simulink model "rmspec"  (Simulink 7.0)
settings: Solver=ode45  StartTime=0.0  StopTime=200  RelTol=1e-3
undefined symbols (not defined in the file): pfb_coeff_gen_calc
libraries: xbsIndex_r4 x3092, casper_library x230, xps_library x24
(part 20 of 33)

== system rmspec/pfb/fft_wideband_real1/fft_direct/butterfly1_1/twiddle/coeff_gen ==
  rst : Inport
  Counter : xbsIndex_r4/Counter  cnt_type=Free Running  cnt_to=Inf  operation=Up  start_count=0  cnt_by_val=1  arith_type=Unsigned  n_bits=9  bin_pt=0  load_pin=off  rst=on  en=off  explicit_period=on  period=1  dbl_ovrd=off  use_behavioral_HDL=off  use_rpm=off  implementation=Fabric  block_type=counter
  ROM : xbsIndex_r4/ROM  depth=512  initVector=[1 0.999984741210938 0.999923706054688 0.999832153320313 0.999702453613281 0.999526977539063 0.999320983886719 0.999076843261719 0.998794555664063 0.99847412109375 0.998115539550781 0.997726440429688 0.997291564941406 0.996818542480469 0.996315002441406 0.995765686035156 0.995185852050781 0.99456787109375 0.993904113769531 0.993209838867188 0.992477416992188 0.991706848144531 0.99090576171875 0.990058898925781 0.989173889160156 0.988258361816406 0.9873046875 0.986305236816406 0.985275268554688 0.984207153320313 0.983108520507813 0.981964111328125 0.980781555175781 0.979568481445313 0.978317260742188 0.977027893066406 0.975700378417969 0.974342346191406 0.972938537597656 0.971504211425781 0.97003173828125 0.968521118164063 0.96697998046875 0.96539306640625 0.963775634765625 0.962120056152344 0.960433959960938 0.958702087402344 0.956939697265625 0.95513916015625 0.95330810546875 0.951431274414063 0.949531555175781 0.947586059570313 0.945610046386719 0.943595886230469 0.941543579101563 0.939460754394531 0.937339782714844 0.9351806640625 0.932991027832031 0.930763244628906 0.928504943847656 0.92620849609375 0.923881530761719 0.921516418457031 0.919113159179688 0.916679382324219 0.914207458496094 0.911705017089844 0.909164428710938 0.906593322753906 0.90399169921875 0.901351928710938 0.898674011230469 0.895965576171875 0.893226623535156 0.890449523925781 0.887641906738281 0.884796142578125 0.881919860839844 0.879013061523438 0.876068115234375 0.873092651367188 0.870086669921875 0.867042541503906 0.863975524902344 0.860870361328125 0.85772705078125 0.854560852050781 0.851356506347656 0.848121643066406 0.844856262207031 0.841552734375 0.838226318359375 0.834861755371094 0.831466674804688 0.828048706054688 0.824592590332031 0.82110595703125 0.817581176757813 0.814033508300781 0.810455322265625 0.806846618652344 0.803207397460938 0.799537658691406 0.79583740234375 0.792106628417969 0.788345336914063 0.784553527832031 0.780738830566406 0.776885986328125 0.77301025390625 0.76910400390625 0.765167236328125 0.761199951171875 0.757209777832031 0.753189086914063 0.749137878417969 0.74505615234375 0.740951538085938 0.73681640625 0.732650756835938 0.728462219238281 0.724250793457031 0.720001220703125 0.715728759765625 0.711433410644531 0.707107543945313 0.702751159667969 0.698379516601563 0.6939697265625 0.689537048339844 0.685081481933594 0.68060302734375 0.676094055175781 0.671562194824219 0.666999816894531 0.66241455078125 0.657806396484375 0.653175354003906 0.648513793945313 0.643829345703125 0.639122009277344 0.634391784667969 0.629638671875 0.624862670898438 0.62005615234375 0.615234375 0.610382080078125 0.605514526367188 0.600616455078125 0.595695495605469 0.59075927734375 0.585800170898438 0.580810546875 0.5758056640625 0.570777893066406 0.56573486328125 0.560661315917969 0.555572509765625 0.550460815429688 0.545326232910156 0.540168762207031 0.534996032714844 0.529800415039063 0.524589538574219 0.519355773925781 0.51409912109375 0.508827209472656 0.5035400390625 0.49822998046875 0.492897033691406 0.487548828125 0.482185363769531 0.476799011230469 0.471397399902344 0.465972900390625 0.460540771484375 0.455085754394531 0.449607849121094 0.444122314453125 0.438613891601563 0.433090209960938 0.427558898925781 0.4219970703125 0.416427612304688 0.410842895507813 0.405242919921875 0.399627685546875 0.393989562988281 0.388343811035156 0.382682800292969 0.377006530761719 0.371315002441406 0.365615844726563 0.359893798828125 0.354164123535156 0.348419189453125 0.342658996582031 0.336891174316406 0.331108093261719 0.325309753417969 0.319503784179688 0.313682556152344 0.307846069335938 0.302009582519531 0.296150207519531 0.290283203125 0.284408569335938 0.278518676757813 0.272621154785156 0.266716003417969 0.260795593261719 0.254867553710938 0.248924255371094 0.24298095703125 0.237022399902344 0.231056213378906 0.225082397460938 0.219100952148438 0.213111877441406 0.207115173339844 0.201103210449219 0.195091247558594 0.189071655273438 ...(+5321 chars)]  distributed_mem=Block RAM  rst=off  init_reg=0  en=off  latency=2  arith_type="Signed  (2's comp)"  n_bits=18  bin_pt=17  dbl_ovrd=off  optimize=Area  use_rpm=on  block_type=sprom
      settings: block_version=10.1.3
  ROM1 : xbsIndex_r4/ROM  depth=512  initVector=[0 -0.006134033203125 -0.01226806640625 -0.0184097290039063 -0.0245437622070313 -0.0306777954101563 -0.03680419921875 -0.042938232421875 -0.0490646362304688 -0.0551986694335938 -0.0613174438476563 -0.06744384765625 -0.0735626220703125 -0.079681396484375 -0.0858001708984375 -0.0919113159179688 -0.0980148315429688 -0.104118347167969 -0.110221862792969 -0.116317749023438 -0.122413635253906 -0.128501892089844 -0.13458251953125 -0.140655517578125 -0.146728515625 -0.152793884277344 -0.158859252929688 -0.164909362792969 -0.17095947265625 -0.177001953125 -0.183036804199219 -0.189071655273438 -0.195091247558594 -0.201103210449219 -0.207115173339844 -0.213111877441406 -0.219100952148438 -0.225082397460938 -0.231056213378906 -0.237022399902344 -0.24298095703125 -0.248924255371094 -0.254867553710938 -0.260795593261719 -0.266716003417969 -0.272621154785156 -0.278518676757813 -0.284408569335938 -0.290283203125 -0.296150207519531 -0.302009582519531 -0.307846069335938 -0.313682556152344 -0.319503784179688 -0.325309753417969 -0.331108093261719 -0.336891174316406 -0.342658996582031 -0.348419189453125 -0.354164123535156 -0.359893798828125 -0.365615844726563 -0.371315002441406 -0.377006530761719 -0.382682800292969 -0.388343811035156 -0.393989562988281 -0.399627685546875 -0.405242919921875 -0.410842895507813 -0.416427612304688 -0.4219970703125 -0.427558898925781 -0.433090209960938 -0.438613891601563 -0.444122314453125 -0.449607849121094 -0.455085754394531 -0.460540771484375 -0.465972900390625 -0.471397399902344 -0.476799011230469 -0.482185363769531 -0.487548828125 -0.492897033691406 -0.49822998046875 -0.5035400390625 -0.508827209472656 -0.51409912109375 -0.519355773925781 -0.524589538574219 -0.529800415039063 -0.534996032714844 -0.540168762207031 -0.545326232910156 -0.550460815429688 -0.555572509765625 -0.560661315917969 -0.56573486328125 -0.570777893066406 -0.5758056640625 -0.580810546875 -0.585800170898438 -0.59075927734375 -0.595695495605469 -0.600616455078125 -0.605514526367188 -0.610382080078125 -0.615234375 -0.62005615234375 -0.624862670898438 -0.629638671875 -0.634391784667969 -0.639122009277344 -0.643829345703125 -0.648513793945313 -0.653175354003906 -0.657806396484375 -0.66241455078125 -0.666999816894531 -0.671562194824219 -0.676094055175781 -0.68060302734375 -0.685081481933594 -0.689537048339844 -0.6939697265625 -0.698379516601563 -0.702751159667969 -0.707107543945313 -0.711433410644531 -0.715728759765625 -0.720001220703125 -0.724250793457031 -0.728462219238281 -0.732650756835938 -0.73681640625 -0.740951538085938 -0.74505615234375 -0.749137878417969 -0.753189086914063 -0.757209777832031 -0.761199951171875 -0.765167236328125 -0.76910400390625 -0.77301025390625 -0.776885986328125 -0.780738830566406 -0.784553527832031 -0.788345336914063 -0.792106628417969 -0.79583740234375 -0.799537658691406 -0.803207397460938 -0.806846618652344 -0.810455322265625 -0.814033508300781 -0.817581176757813 -0.82110595703125 -0.824592590332031 -0.828048706054688 -0.831466674804688 -0.834861755371094 -0.838226318359375 -0.841552734375 -0.844856262207031 -0.848121643066406 -0.851356506347656 -0.854560852050781 -0.85772705078125 -0.860870361328125 -0.863975524902344 -0.867042541503906 -0.870086669921875 -0.873092651367188 -0.876068115234375 -0.879013061523438 -0.881919860839844 -0.884796142578125 -0.887641906738281 -0.890449523925781 -0.893226623535156 -0.895965576171875 -0.898674011230469 -0.901351928710938 -0.90399169921875 -0.906593322753906 -0.909164428710938 -0.911705017089844 -0.914207458496094 -0.916679382324219 -0.919113159179688 -0.921516418457031 -0.923881530761719 -0.92620849609375 -0.928504943847656 -0.930763244628906 -0.932991027832031 -0.9351806640625 -0.937339782714844 -0.939460754394531 -0.941543579101563 -0.943595886230469 -0.945610046386719 -0.947586059570313 -0.949531555175781 -0.951431274414063 -0.95330810546875 -0.95513916015625 -0.956939697265625 -0.958702087402344 -0.960433959960938 -0.962120056152344 -0.963775634765625 -0.96539306640625 ...(+5571 chars)]  distributed_mem=Block RAM  rst=off  init_reg=0  en=off  latency=2  arith_type="Signed  (2's comp)"  n_bits=18  bin_pt=17  dbl_ovrd=off  optimize=Area  use_rpm=on  block_type=sprom
      settings: block_version=10.1.3
  Slice : xbsIndex_r4/Slice  nbits=9  boolean_output=off  mode=Upper Bit Location + Width  bit1=0  base1=MSB of Input  bit0=0  base0=LSB of Input  dbl_ovrd=off  block_type=slice
      settings: infoedit="Extracts a given range of bits from each input sample and presents it at the output.  The output type is ordinarily unsigned with binary point at zero, but can be Boolean when the slice is one bit wide.<P><P>Hardware notes: In hardware this block costs nothing."  block_version=10.1.3
  ri_to_c : casper_library/Misc/ri_to_c  SystemSampleTime=-1
  w : Outport
  wires:
  ri_to_c/1 -> w/1
  rst/1 -> Counter/1
  Counter/1 -> Slice/1
  Slice/1 -> ROM/1, ROM1/1
  ROM/1 -> ri_to_c/1
  ROM1/1 -> ri_to_c/2

== system rmspec/pfb/fft_wideband_real1/fft_direct/butterfly1_1/twiddle/convert_of ==
  din : Inport  OutDataType=sfix(16)  OutScaling=2^0
  convert : xbsIndex_r4/Convert  arith_type="Signed  (2's comp)"  n_bits=bit_width_o  bin_pt=binary_point_o  quantization=Truncate  overflow=Wrap  latency=latency  dbl_ovrd=off  pipeline=on  block_type=convert
      settings: block_version=10.1.1
  never : xbsIndex_r4/Constant  arith_type=Boolean  const=0  n_bits=16  bin_pt=14  explicit_period=on  period=1  equ=P=C  opselect=C  inp2=PCIN>>17  opr=+  inp1=P  carry=CIN  dbl_ovrd=off  block_type=constant
  dout : Outport
  of : Outport  Port=2
  wires:
  din/1 -> convert/1
  convert/1 -> dout/1
  never/1 -> of/1

== system rmspec/pfb/fft_wideband_real1/fft_direct/butterfly1_1/twiddle/convert_of1 ==
  din : Inport  OutDataType=sfix(16)  OutScaling=2^0
  convert : xbsIndex_r4/Convert  arith_type="Signed  (2's comp)"  n_bits=bit_width_o  bin_pt=binary_point_o  quantization=Truncate  overflow=Wrap  latency=latency  dbl_ovrd=off  pipeline=on  block_type=convert
      settings: block_version=10.1.1
  never : xbsIndex_r4/Constant  arith_type=Boolean  const=0  n_bits=16  bin_pt=14  explicit_period=on  period=1  equ=P=C  opselect=C  inp2=PCIN>>17  opr=+  inp1=P  carry=CIN  dbl_ovrd=off  block_type=constant
  dout : Outport
  of : Outport  Port=2
  wires:
  din/1 -> convert/1
  convert/1 -> dout/1
  never/1 -> of/1

== system rmspec/pfb/fft_wideband_real1/fft_direct/butterfly2_0/twiddle/coeff_gen ==
  rst : Inport
  Counter : xbsIndex_r4/Counter  cnt_type=Free Running  cnt_to=Inf  operation=Up  start_count=0  cnt_by_val=1  arith_type=Unsigned  n_bits=9  bin_pt=0  load_pin=off  rst=on  en=off  explicit_period=on  period=1  dbl_ovrd=off  use_behavioral_HDL=off  use_rpm=off  implementation=Fabric  block_type=counter
  ROM : xbsIndex_r4/ROM  depth=512  initVector=[1 0.999992370605469 0.999984741210938 0.999954223632813 0.999923706054688 0.999885559082031 0.999832153320313 0.999771118164063 0.999702453613281 0.999618530273438 0.999526977539063 0.999427795410156 0.999320983886719 0.99920654296875 0.999076843261719 0.998939514160156 0.998794555664063 0.998641967773438 0.99847412109375 0.998298645019531 0.998115539550781 0.9979248046875 0.997726440429688 0.997512817382813 0.997291564941406 0.997062683105469 0.996818542480469 0.996574401855469 0.996315002441406 0.996047973632813 0.995765686035156 0.9954833984375 0.995185852050781 0.994880676269531 0.99456787109375 0.994239807128906 0.993904113769531 0.993560791015625 0.993209838867188 0.992851257324219 0.992477416992188 0.992095947265625 0.991706848144531 0.991310119628906 0.99090576171875 0.990486145019531 0.990058898925781 0.9896240234375 0.989173889160156 0.988723754882813 0.988258361816406 0.987785339355469 0.9873046875 0.986808776855469 0.986305236816406 0.985794067382813 0.985275268554688 0.984748840332031 0.984207153320313 0.983665466308594 0.983108520507813 0.982536315917969 0.981964111328125 0.981376647949219 0.980781555175781 0.980178833007813 0.979568481445313 0.978950500488281 0.978317260742188 0.977676391601563 0.977027893066406 0.976371765136719 0.975700378417969 0.975028991699219 0.974342346191406 0.973640441894531 0.972938537597656 0.97222900390625 0.971504211425781 0.970771789550781 0.97003173828125 0.969284057617188 0.968521118164063 0.967750549316406 0.96697998046875 0.9661865234375 0.96539306640625 0.964591979980469 0.963775634765625 0.96295166015625 0.962120056152344 0.961280822753906 0.960433959960938 0.959571838378906 0.958702087402344 0.95782470703125 0.956939697265625 0.956047058105469 0.95513916015625 0.954231262207031 0.95330810546875 0.952377319335938 0.951431274414063 0.950485229492188 0.949531555175781 0.948562622070313 0.947586059570313 0.946601867675781 0.945610046386719 0.944602966308594 0.943595886230469 0.942573547363281 0.941543579101563 0.940505981445313 0.939460754394531 0.938400268554688 0.937339782714844 0.936264038085938 0.9351806640625 0.934089660644531 0.932991027832031 0.931884765625 0.930763244628906 0.929641723632813 0.928504943847656 0.927360534667969 0.92620849609375 0.925048828125 0.923881530761719 0.922698974609375 0.921516418457031 0.920318603515625 0.919113159179688 0.917900085449219 0.916679382324219 0.915451049804688 0.914207458496094 0.9129638671875 0.911705017089844 0.910438537597656 0.909164428710938 0.907882690429688 0.906593322753906 0.905296325683594 0.90399169921875 0.902671813964844 0.901351928710938 0.900016784667969 0.898674011230469 0.897323608398438 0.895965576171875 0.894599914550781 0.893226623535156 0.891838073730469 0.890449523925781 0.889045715332031 0.887641906738281 0.886222839355469 0.884796142578125 0.88336181640625 0.881919860839844 0.880470275878906 0.879013061523438 0.877548217773438 0.876068115234375 0.874588012695313 0.873092651367188 0.871597290039063 0.870086669921875 0.868568420410156 0.867042541503906 0.865516662597656 0.863975524902344 0.8624267578125 0.860870361328125 0.859298706054688 0.85772705078125 0.856147766113281 0.854560852050781 0.852958679199219 0.851356506347656 0.849739074707031 0.848121643066406 0.846488952636719 0.844856262207031 0.843208312988281 0.841552734375 0.839897155761719 0.838226318359375 0.8365478515625 0.834861755371094 0.833168029785156 0.831466674804688 0.829757690429688 0.828048706054688 0.826324462890625 0.824592590332031 0.822853088378906 0.82110595703125 0.819351196289063 0.817581176757813 0.815811157226563 0.814033508300781 0.812248229980469 0.810455322265625 0.80865478515625 0.806846618652344 0.805030822753906 0.803207397460938 0.801376342773438 0.799537658691406 0.797691345214844 0.79583740234375 0.793975830078125 0.792106628417969 0.790229797363281 0.788345336914063 0.786453247070313 0.784553527832031 0.78265380859375 0.780738830566406 0.778816223144531 0.776885986328125 0.774955749511719 0.77301025390625 ...(+5107 chars)]  distributed_mem=Block RAM  rst=off  init_reg=0  en=off  latency=2  arith_type="Signed  (2's comp)"  n_bits=18  bin_pt=17  dbl_ovrd=off  optimize=Area  use_rpm=on  block_type=sprom
      settings: block_version=10.1.3
  ROM1 : xbsIndex_r4/ROM  depth=512  initVector=[0 -0.0030670166015625 -0.006134033203125 -0.0092010498046875 -0.01226806640625 -0.0153427124023438 -0.0184097290039063 -0.0214767456054688 -0.0245437622070313 -0.0276107788085938 -0.0306777954101563 -0.0337448120117188 -0.03680419921875 -0.0398712158203125 -0.042938232421875 -0.0460052490234375 -0.0490646362304688 -0.0521316528320313 -0.0551986694335938 -0.058258056640625 -0.0613174438476563 -0.0643844604492188 -0.06744384765625 -0.0705032348632813 -0.0735626220703125 -0.0766220092773438 -0.079681396484375 -0.0827407836914063 -0.0858001708984375 -0.0888519287109375 -0.0919113159179688 -0.0949630737304688 -0.0980148315429688 -0.101066589355469 -0.104118347167969 -0.107170104980469 -0.110221862792969 -0.113273620605469 -0.116317749023438 -0.119361877441406 -0.122413635253906 -0.125457763671875 -0.128501892089844 -0.131538391113281 -0.13458251953125 -0.137619018554688 -0.140655517578125 -0.143692016601563 -0.146728515625 -0.149765014648438 -0.152793884277344 -0.155830383300781 -0.158859252929688 -0.161888122558594 -0.164909362792969 -0.167938232421875 -0.17095947265625 -0.173980712890625 -0.177001953125 -0.180023193359375 -0.183036804199219 -0.186058044433594 -0.189071655273438 -0.19207763671875 -0.195091247558594 -0.198097229003906 -0.201103210449219 -0.204109191894531 -0.207115173339844 -0.210113525390625 -0.213111877441406 -0.216110229492188 -0.219100952148438 -0.222091674804688 -0.225082397460938 -0.228073120117188 -0.231056213378906 -0.234039306640625 -0.237022399902344 -0.240005493164063 -0.24298095703125 -0.245956420898438 -0.248924255371094 -0.251899719238281 -0.254867553710938 -0.257827758789063 -0.260795593261719 -0.263755798339844 -0.266716003417969 -0.269668579101563 -0.272621154785156 -0.27557373046875 -0.278518676757813 -0.281463623046875 -0.284408569335938 -0.287345886230469 -0.290283203125 -0.293220520019531 -0.296150207519531 -0.299079895019531 -0.302009582519531 -0.304931640625 -0.307846069335938 -0.310768127441406 -0.313682556152344 -0.316596984863281 -0.319503784179688 -0.322410583496094 -0.325309753417969 -0.328208923339844 -0.331108093261719 -0.333999633789063 -0.336891174316406 -0.339775085449219 -0.342658996582031 -0.345542907714844 -0.348419189453125 -0.351295471191406 -0.354164123535156 -0.357032775878906 -0.359893798828125 -0.362754821777344 -0.365615844726563 -0.36846923828125 -0.371315002441406 -0.374160766601563 -0.377006530761719 -0.379844665527344 -0.382682800292969 -0.385513305664063 -0.388343811035156 -0.391166687011719 -0.393989562988281 -0.396812438964844 -0.399627685546875 -0.402435302734375 -0.405242919921875 -0.408042907714844 -0.410842895507813 -0.41363525390625 -0.416427612304688 -0.419219970703125 -0.4219970703125 -0.424781799316406 -0.427558898925781 -0.430328369140625 -0.433090209960938 -0.435859680175781 -0.438613891601563 -0.441368103027344 -0.444122314453125 -0.446868896484375 -0.449607849121094 -0.452346801757813 -0.455085754394531 -0.457817077636719 -0.460540771484375 -0.4632568359375 -0.465972900390625 -0.46868896484375 -0.471397399902344 -0.474098205566406 -0.476799011230469 -0.4794921875 -0.482185363769531 -0.484870910644531 -0.487548828125 -0.490226745605469 -0.492897033691406 -0.495567321777344 -0.49822998046875 -0.500885009765625 -0.5035400390625 -0.506187438964844 -0.508827209472656 -0.511466979980469 -0.51409912109375 -0.516731262207031 -0.519355773925781 -0.52197265625 -0.524589538574219 -0.527198791503906 -0.529800415039063 -0.532402038574219 -0.534996032714844 -0.537590026855469 -0.540168762207031 -0.542747497558594 -0.545326232910156 -0.547897338867188 -0.550460815429688 -0.553016662597656 -0.555572509765625 -0.558120727539063 -0.560661315917969 -0.563201904296875 -0.56573486328125 -0.568260192871094 -0.570777893066406 -0.573295593261719 -0.5758056640625 -0.578315734863281 -0.580810546875 -0.583305358886719 -0.585800170898438 -0.588279724121094 -0.59075927734375 -0.593231201171875 -0.595695495605469 -0.598159790039063 -0.600616455078125 -0.603065490722656 ...(+5615 chars)]  distributed_mem=Block RAM  rst=off  init_reg=0  en=off  latency=2  arith_type="Signed  (2's comp)"  n_bits=18  bin_pt=17  dbl_ovrd=off  optimize=Area  use_rpm=on  block_type=sprom
      settings: block_version=10.1.3
  Slice : xbsIndex_r4/Slice  nbits=9  boolean_output=off  mode=Upper Bit Location + Width  bit1=0  base1=MSB of Input  bit0=0  base0=LSB of Input  dbl_ovrd=off  block_type=slice
      settings: infoedit="Extracts a given range of bits from each input sample and presents it at the output.  The output type is ordinarily unsigned with binary point at zero, but can be Boolean when the slice is one bit wide.<P><P>Hardware notes: In hardware this block costs nothing."  block_version=10.1.3
  ri_to_c : casper_library/Misc/ri_to_c  SystemSampleTime=-1
  w : Outport
  wires:
  ri_to_c/1 -> w/1
  rst/1 -> Counter/1
  Counter/1 -> Slice/1
  Slice/1 -> ROM/1, ROM1/1
  ROM/1 -> ri_to_c/1
  ROM1/1 -> ri_to_c/2

== system rmspec/pfb/fft_wideband_real1/fft_direct/butterfly2_0/twiddle/convert_of ==
  din : Inport  OutDataType=sfix(16)  OutScaling=2^0
  convert : xbsIndex_r4/Convert  arith_type="Signed  (2's comp)"  n_bits=bit_width_o  bin_pt=binary_point_o  quantization=Truncate  overflow=Wrap  latency=latency  dbl_ovrd=off  pipeline=on  block_type=convert
      settings: block_version=10.1.1
  never : xbsIndex_r4/Constant  arith_type=Boolean  const=0  n_bits=16  bin_pt=14  explicit_period=on  period=1  equ=P=C  opselect=C  inp2=PCIN>>17  opr=+  inp1=P  carry=CIN  dbl_ovrd=off  block_type=constant
  dout : Outport
  of : Outport  Port=2
  wires:
  din/1 -> convert/1
  convert/1 -> dout/1
  never/1 -> of/1

== system rmspec/pfb/fft_wideband_real1/fft_direct/butterfly2_0/twiddle/convert_of1 ==
  din : Inport  OutDataType=sfix(16)  OutScaling=2^0
  convert : xbsIndex_r4/Convert  arith_type="Signed  (2's comp)"  n_bits=bit_width_o  bin_pt=binary_point_o  quantization=Truncate  overflow=Wrap  latency=latency  dbl_ovrd=off  pipeline=on  block_type=convert
      settings: block_version=10.1.1
  never : xbsIndex_r4/Constant  arith_type=Boolean  const=0  n_bits=16  bin_pt=14  explicit_period=on  period=1  equ=P=C  opselect=C  inp2=PCIN>>17  opr=+  inp1=P  carry=CIN  dbl_ovrd=off  block_type=constant
  dout : Outport
  of : Outport  Port=2
  wires:
  din/1 -> convert/1
  convert/1 -> dout/1
  never/1 -> of/1
